simulink model "FotoTParam"  (R2021b)
settings: Solver=VariableStepAuto  StartTime=-10  StopTime=10  RelTol=1e-3
settings Model: Creator=Siro  LastModifiedBy=david

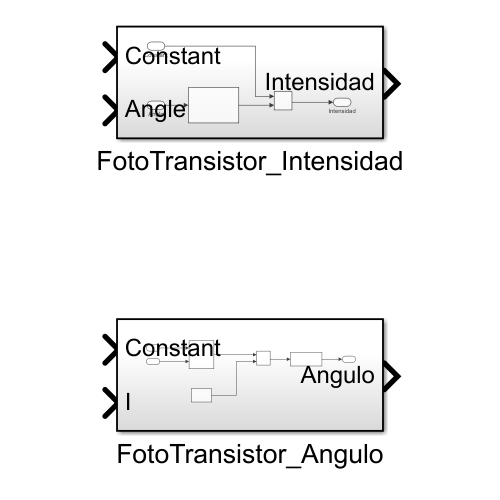
[thumbnail: Simulink's stored preview of the top-level diagram]
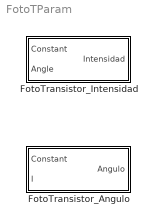
== system FotoTParam ==
  FotoTransistor_Angulo : Subsystem
  FotoTransistor_Intensidad : Subsystem

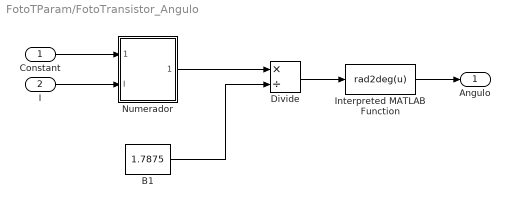
== system FotoTParam/FotoTransistor_Angulo ==
  Constant : Inport
  I : Inport  Port=2
  B1 : Constant  Value=1.7875
  Divide : Product  Inputs=*/
  Interpreted MATLAB Function : MATLABFcn  MATLABFcn=rad2deg(u)
  Numerador : Subsystem
  Angulo : Outport
  wires:
  B1/1 -> Divide/2
  Constant/1 -> Numerador/1(Constant)
  I/1 -> Numerador/2(I)
  Numerador/1(Out1) -> Divide/1
  Divide/1 -> Interpreted MATLAB Function/1
  Interpreted MATLAB Function/1 -> Angulo/1

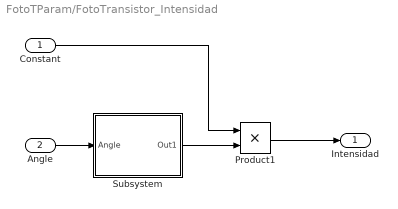
== system FotoTParam/FotoTransistor_Intensidad ==
  Constant : Inport
  Angle : Inport  Port=2
  Product1 : Product
  Subsystem : Subsystem
  Intensidad : Outport
  wires:
  Angle/1 -> Subsystem/1(Angle)
  Constant/1 -> Product1/1
  Subsystem/1(Out1) -> Product1/2
  Product1/1 -> Intensidad/1

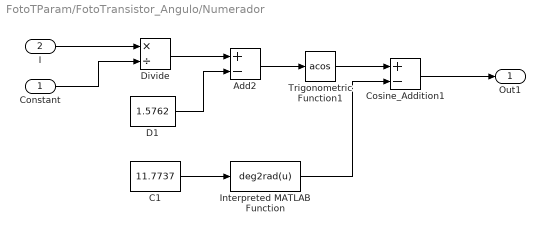
== system FotoTParam/FotoTransistor_Angulo/Numerador ==
  Constant : Inport
  I : Inport  Port=2
  Add2 : Sum  Inputs=+-
  C1 : Constant  Value=11.7737
  Cosine_Addition1 : Sum  Inputs=+-
  D1 : Constant  Value=1.5762
  Divide : Product  Inputs=*/
  Interpreted MATLAB Function : MATLABFcn  MATLABFcn=deg2rad(u)
  Trigonometric Function1 : Trigonometry  Operator=acos
  Out1 : Outport
  wires:
  Trigonometric Function1/1 -> Cosine_Addition1/1
  C1/1 -> Interpreted MATLAB Function/1
  Cosine_Addition1/1 -> Out1/1
  Interpreted MATLAB Function/1 -> Cosine_Addition1/2
  D1/1 -> Add2/2
  Divide/1 -> Add2/1
  Add2/1 -> Trigonometric Function1/1
  I/1 -> Divide/1
  Constant/1 -> Divide/2

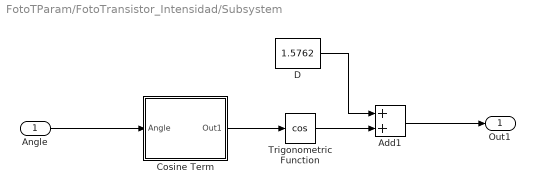
== system FotoTParam/FotoTransistor_Intensidad/Subsystem ==
  Angle : Inport
  Add1 : Sum
  Cosine Term : Subsystem
  D : Constant  Value=1.5762
  Trigonometric Function : Trigonometry  Operator=cos
  Out1 : Outport
  wires:
  Cosine Term/1(Out1) -> Trigonometric Function/1
  Angle/1 -> Cosine Term/1(Angle)
  Add1/1 -> Out1/1
  Trigonometric Function/1 -> Add1/2
  D/1 -> Add1/1

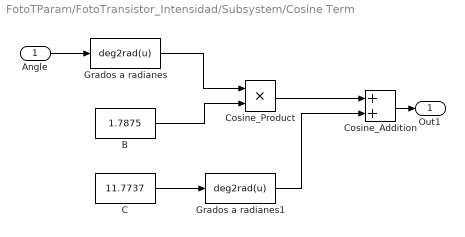
== system FotoTParam/FotoTransistor_Intensidad/Subsystem/Cosine Term ==
  Angle : Inport
  B : Constant  Value=1.7875
  C : Constant  Value=11.7737
  Cosine_Addition : Sum
  Cosine_Product : Product
  Grados a radianes : MATLABFcn  MATLABFcn=deg2rad(u)
  Grados a radianes1 : MATLABFcn  MATLABFcn=deg2rad(u)
  Out1 : Outport
  wires:
  Angle/1 -> Grados a radianes/1
  B/1 -> Cosine_Product/2
  Cosine_Product/1 -> Cosine_Addition/1
  Cosine_Addition/1 -> Out1/1
  C/1 -> Grados a radianes1/1
  Grados a radianes/1 -> Cosine_Product/1
  Grados a radianes1/1 -> Cosine_Addition/2
